simulink model "doc_convcoding"  (R2014a)
settings: Solver=ode45  StartTime=0.0  StopTime=inf  RelTol=1e-3
undefined symbols (not defined in the file or in its folder): commblksprivate, Info
libraries: commcnvcod2 x2, commrandsrc2 x1, commchan3 x1, commsink2 x1
settings Model: Creator=The MathWorks Inc.
settings DataIOCC: SignalLoggingSaveFormat=ModelDataLogs  SignalLoggingName=sigsOut
settings OptimizationCC: BlockReduction=off  BooleanDataType=off  ExpressionDepthLimit=2147483647
settings DebuggingCC: SaveWithParameterizedLinksMsg=none  UnderspecifiedInitializationDetection=Classic  SolverPrmCheckMsg=none  MultiTaskDSMMsg=warning  MultiTaskCondExecSysMsg=none  FcnCallInpInsideContextMsg=UseLocalSettings  StateNameClashWarn=warning  StrictBusMsg=None
settings HardwareCC: ProdHWDeviceType=Specified
settings RTWCC: IncludeERTFirstTime=on
settings GRTTargetCC: TargetFcnLib=iso_c_tmw.mat  CombineOutputUpdateFcns=off  GRTInterface=on

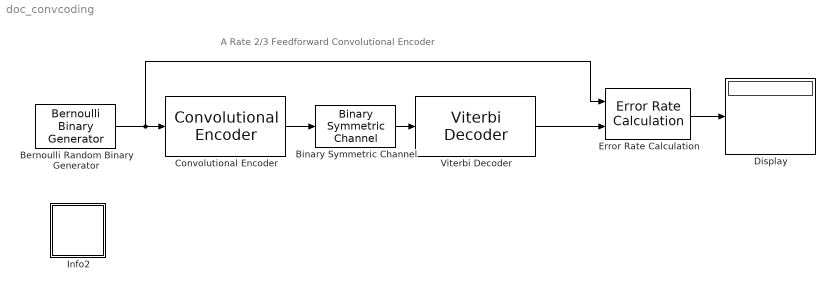
== system doc_convcoding ==
  note: A Rate 2/3 Feedforward Convolutional Encoder
  Bernoulli Random Binary Generator : commrandsrc2/Bernoulli Binary Generator  P=.5  seed=129499  Ts=.5  frameBased=on  sampPerFrame=2  orient=off  outDataType=double
  Binary Symmetric Channel : commchan3/Binary Symmetric Channel  P=0.02  s=149  E=off  outDtype=double
  Convolutional Encoder : commcnvcod2/Convolutional Encoder  trellis=poly2trellis([5 4], [23 35 0; 0 5 13] )  opMode=Continuous  DelayedResetAction=off  hasIniStPort=off  hasFinStPort=off  usePuncVector=off  punctureVector=[1; 1; 0; 1; 0; 1]  reset=Unused parameter value
  Display : Display
  Error Rate Calculation : commsink2/Error Rate Calculation  N=68  st_delay=0  cp_mode=Entire frame  subframe=[]  PMode=Port  WsName=ErrorVec  RsMode2=off  stop=on  numErr=100  maxBits=1e6
  Info2 : Subsystem  AncestorBlock=commblksprivate/Info  mask(Info){}
      settings: OpenFcn=helpview([docroot '/toolbox/comm/comm.map'], 'doc_convcoding')
      mask Display: disp('Info')
  Viterbi Decoder : commcnvcod2/Viterbi Decoder  trellis=poly2trellis([5 4], [23 35 0; 0 5 13] )  isPunctured=off  punctureVector=[1; 1; 0; 1; 0; 1]  erasures=off  dectype=Hard decision  runSigValErrCheck=off  nsdecb=4  smWordLength=16  tbdepth=34  opmode=Continuous  reset=off  outDataType=Inherit via internal rule  delayedResetAction=off
  wires:
  Convolutional Encoder/1 -> Binary Symmetric Channel/1
  Binary Symmetric Channel/1 -> Viterbi Decoder/1
  Error Rate Calculation/1 -> Display/1
  Bernoulli Random Binary Generator/1 -> Convolutional Encoder/1, Error Rate Calculation/1
  Viterbi Decoder/1 -> Error Rate Calculation/2

== system doc_convcoding/Info2 ==
